simulink model "PWM"  (R2022a)
settings: Solver=FixedStepAuto  StartTime=0.0  StopTime=inf  FixedStep=0.005  RelTol=1e-3  EnableMultiTasking=on
libraries: arduinolib x5
settings Model: ExtModeTrigDuration=2  Creator=user  LastModifiedBy=user
settings OptimizationCC: EnhancedBackFolding=on  PassReuseOutputArgsAs=Individual arguments  ZeroExternalMemoryAtStartup=off  ZeroInternalMemoryAtStartup=off  MaxStackSize=64  OptimizeBlockOrder=speed  DifferentSizesBufferReuse=on  OptimizationCustomize=off  EfficientTunableParamExpr=on
settings DebuggingCC: ParameterTunabilityLossMsg=error
settings HardwareCC: ProdBitPerPointer=32  ProdBitPerSizeT=32  ProdBitPerPtrDiffT=32  ProdLargestAtomicInteger=Long  ProdLargestAtomicFloat=Double  ProdWordSize=32  ProdHWDeviceType=ARM Compatible->ARM Cortex
settings SFSimCC: MATLABDynamicMemAlloc=off
settings RTWCC: SystemTargetFile=ert.tlc  HardwareBoard=Arduino Due  TemplateMakefile=ert_default_tmf  Toolchain=Arduino ARM  BuildConfiguration=Faster Runs
settings CodeAppCC: ForceParamTrailComments=on  IgnoreCustomStorageClasses=off  OperatorAnnotations=on  SimulinkDataObjDesc=on  SFDataObjDesc=on  InsertBlockDesc=on
settings ERTTargetCC: SupportContinuousTime=on  SupportVariableSizeSignals=on  ExtModeTransport=3  ExtModeStaticAlloc=on  ExtModeStaticAllocSize=24576  ExtModeMexFile=ext_xcp  ExtModeIntrfLevel=Level2 - Open

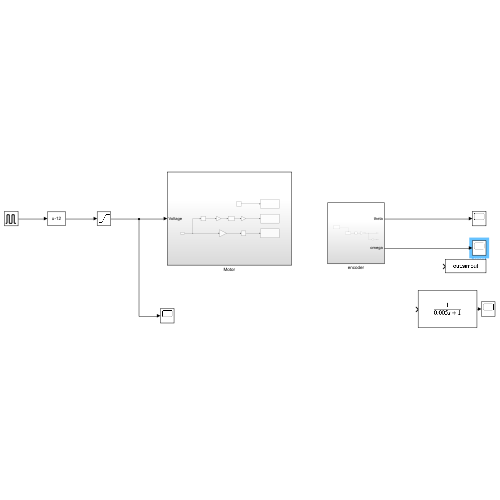
[thumbnail: Simulink's stored preview of the top-level diagram]
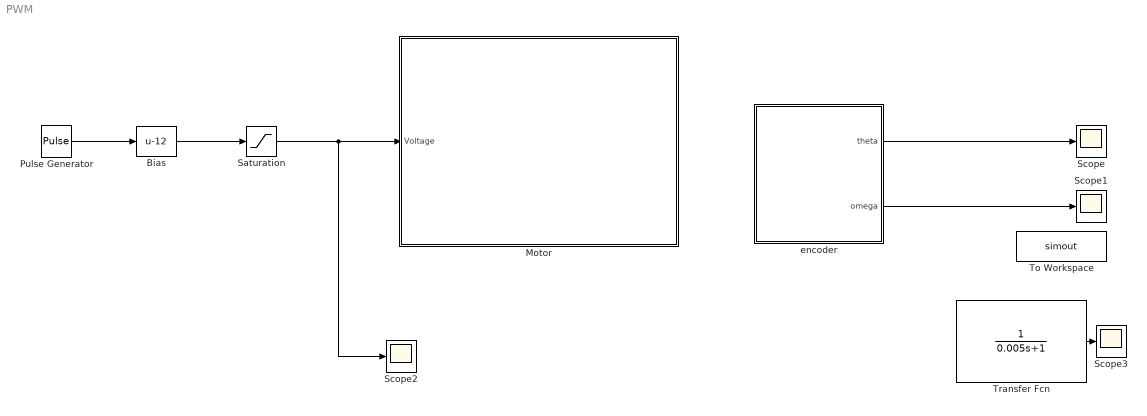
== system PWM ==
  Bias : Bias  Bias=-12  SaturateOnIntegerOverflow=off
  Motor : Subsystem
  Pulse Generator : DiscretePulseGenerator  PulseType=Time based  Amplitude=24  PulseWidth=50
  Saturation : Saturate  UpperLimit=12  LowerLimit=-12
  Scope{,1..3} (4 alike) : Scope
  To Workspace : ToWorkspace  VariableName=simout  SaveFormat=Structure With Time  SampleTime=-1
  Transfer Fcn : TransferFcn  Denominator=[0.005 1]
  encoder : Subsystem
  wires:
  encoder/1(theta) -> Scope/1
  encoder/2(omega) -> Scope1/1
  Saturation/1 -> Scope2/1, Motor/1(Voltage)
  Transfer Fcn/1 -> Scope3/1
  Pulse Generator/1 -> Bias/1
  Bias/1 -> Saturation/1

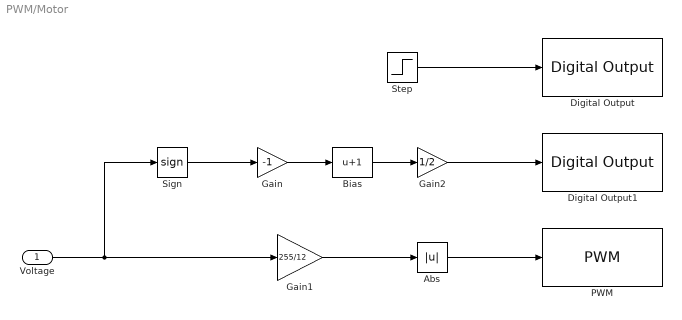
== system PWM/Motor ==
  Voltage : Inport
  Abs : Abs  SaturateOnIntegerOverflow=off
  Bias : Bias  Bias=1  SaturateOnIntegerOverflow=off
  Digital Output : arduinolib/Digital Output  pinNumber=48  Direction=output  blockPlatform=arduino
  Digital Output1 : arduinolib/Digital Output  pinNumber=49  Direction=output  blockPlatform=arduino
  Gain : Gain  Gain=-1
  Gain1 : Gain  Gain=255/12
  Gain2 : Gain  Gain=1/2
  PWM : arduinolib/PWM  pinNumber=2  frequencyType=Default  desiredFrequency=490.2  achievableFrequency=490.2
  Sign : Signum
  Step : Step  Time=5  Before=1  After=0  SampleTime=0
  wires:
  Bias/1 -> Gain2/1
  Step/1 -> Digital Output/1
  Gain1/1 -> Abs/1
  Gain2/1 -> Digital Output1/1
  Voltage/1 -> Sign/1, Gain1/1
  Sign/1 -> Gain/1
  Abs/1 -> PWM/1
  Gain/1 -> Bias/1

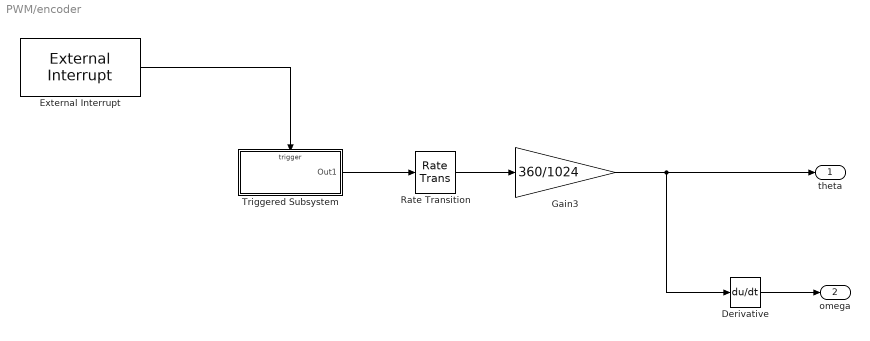
== system PWM/encoder ==
  Derivative : Derivative
  External Interrupt : arduinolib/External Interrupt  Pin=50  PullUp=off  Mode=RISING  InterruptSimulationInput=off
      settings: SourceProductBaseCode=ARDUINO
  Gain3 : Gain  Gain=360/1024
  Rate Transition : RateTransition  Deterministic=off
  Triggered Subsystem : Subsystem  TreatAsAtomicUnit=on
  theta : Outport
  omega : Outport  Port=2
  wires:
  External Interrupt/1 -> Triggered Subsystem/Trigger
  Derivative/1 -> omega/1
  Rate Transition/1 -> Gain3/1
  Triggered Subsystem/1(Out1) -> Rate Transition/1
  Gain3/1 -> theta/1, Derivative/1

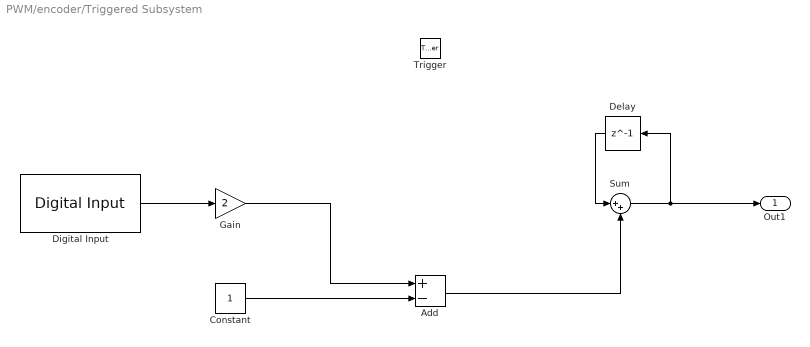
== system PWM/encoder/Triggered Subsystem ==
  Trigger : TriggerPort  TriggerType=function-call  VariantControl=(inherit)
  Add : Sum  Inputs=+-
  Constant : Constant
  Delay : Delay  DelayLength=1
  Digital Input : arduinolib/Digital Input  pinNumber=51  mode=Default  Direction=input  SampleTime=-1  blockPlatform=arduino
  Gain : Gain  Gain=2
  Sum : Sum  Inputs=|++
  Out1 : Outport
  wires:
  Digital Input/1 -> Gain/1
  Constant/1 -> Add/2
  Gain/1 -> Add/1
  Sum/1 -> Out1/1, Delay/1
  Delay/1 -> Sum/1
  Add/1 -> Sum/2
